simulink model "mpc1_simulation"  (R2022b)
settings: Solver=VariableStepAuto  StartTime=0.0  StopTime=T  RelTol=1e-5
undefined symbols (not defined in the file): Am, Bm, c_1, c_2, C_hilf, Cm, D, dt, F1, H1, PhiU1, PhiZ1, Qy1
settings Model: Creator=benja  LastModifiedBy=benja

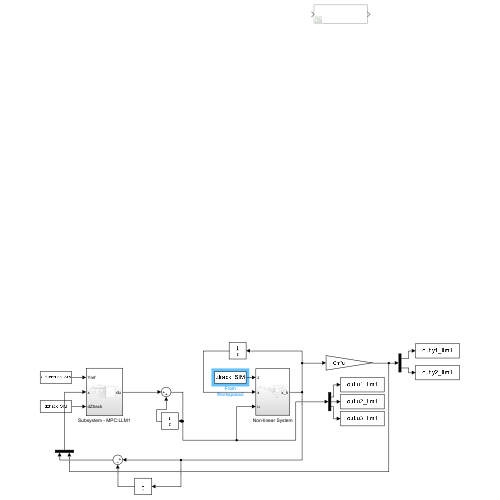
[thumbnail: Simulink's stored preview of the top-level diagram]
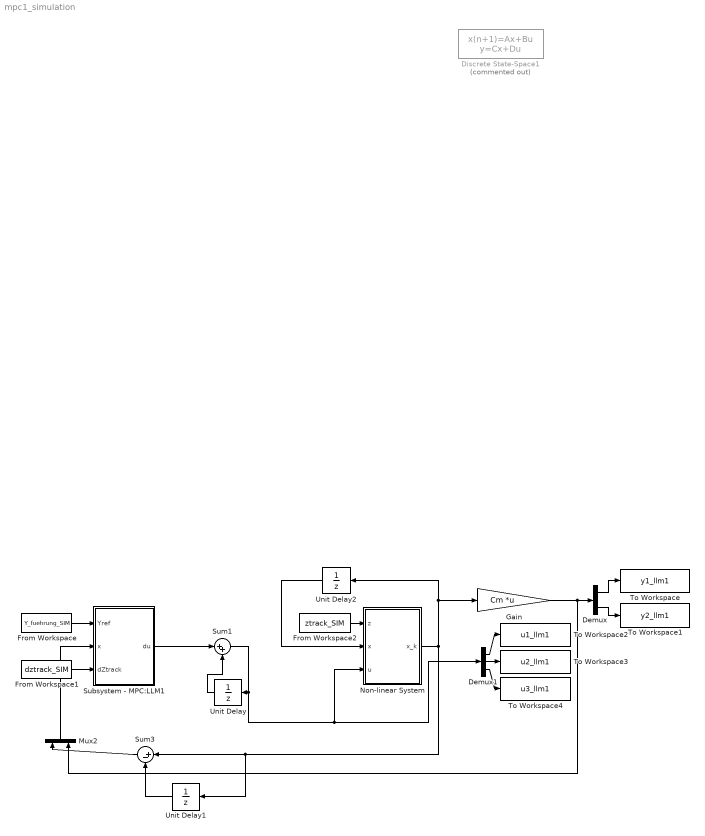
== system mpc1_simulation ==
  Demux : Demux  Outputs=2
  Demux1 : Demux  Outputs=3
  Discrete State-Space1 : DiscreteStateSpace  Commented=on  A=Am  B=Bm  C=C_hilf  D=D  SampleTime=dt
  From Workspace : FromWorkspace  VariableName=Y_fuehrung_SIM  OutDataTypeStr=double  SampleTime=dt
  From Workspace1 : FromWorkspace  VariableName=dztrack_SIM  OutDataTypeStr=double  SampleTime=dt
  From Workspace2 : FromWorkspace  VariableName=ztrack_SIM  OutDataTypeStr=double  SampleTime=dt
  Gain : Gain  Gain=Cm  Multiplication=Matrix(K*u)
  Mux2 : Mux  Inputs=2
  Non-linear System : Subsystem
  Subsystem - MPC:LLM1 : Subsystem
  Sum1 : Sum  Inputs=|++
  Sum3 : Sum  Inputs=|+-
  To Workspace : ToWorkspace  VariableName=y1_llm1  SampleTime=-1
      settings: Save2DSignal=2-D array (concatenate along first dimension)
  To Workspace1 : ToWorkspace  VariableName=y2_llm1  SampleTime=-1
      settings: Save2DSignal=2-D array (concatenate along first dimension)
  To Workspace2 : ToWorkspace  VariableName=u1_llm1  SampleTime=-1
      settings: Save2DSignal=2-D array (concatenate along first dimension)
  To Workspace3 : ToWorkspace  VariableName=u2_llm1  SampleTime=-1
      settings: Save2DSignal=2-D array (concatenate along first dimension)
  To Workspace4 : ToWorkspace  VariableName=u3_llm1  SampleTime=-1
      settings: Save2DSignal=2-D array (concatenate along first dimension)
  Unit Delay : UnitDelay  SampleTime=dt  HasFrameUpgradeWarning=on
  Unit Delay1 : UnitDelay  SampleTime=-1  HasFrameUpgradeWarning=on
  Unit Delay2 : UnitDelay  SampleTime=-1  HasFrameUpgradeWarning=on
  wires:
  Demux/1 -> To Workspace/1
  Demux1/1 -> To Workspace2/1
  Demux1/2 -> To Workspace3/1
  Unit Delay1/1 -> Sum3/2
  Gain/1 -> Demux/1, Mux2/2
  Sum3/1 -> Mux2/1
  Demux1/3 -> To Workspace4/1
  Non-linear System/1(x_k) -> Unit Delay2/1, Gain/1, Unit Delay1/1, Sum3/1
  From Workspace2/1 -> Non-linear System/1(z)
  Unit Delay2/1 -> Non-linear System/2(x)
  Sum1/1 -> Unit Delay/1, Demux1/1, Non-linear System/3(u)
  From Workspace/1 -> Subsystem - MPC:LLM1/1(Yref)
  Mux2/1 -> Subsystem - MPC:LLM1/2(x)
  Demux/2 -> To Workspace1/1
  Unit Delay/1 -> Sum1/2
  From Workspace1/1 -> Subsystem - MPC:LLM1/3(dZtrack)
  Subsystem - MPC:LLM1/1(du) -> Sum1/1

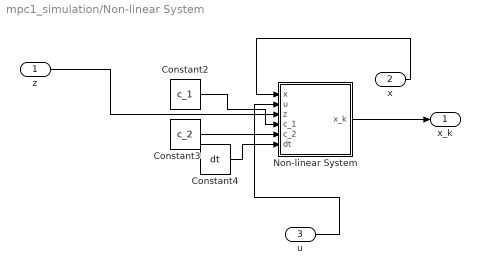
== system mpc1_simulation/Non-linear System ==
  z : Inport
  x : Inport  Port=2
  u : Inport  Port=3
  Constant2 : Constant  Value=c_1
  Constant3 : Constant  Value=c_2
  Constant4 : Constant  Value=dt
  Non-linear System : MATLAB Function  TreatAsAtomicUnit=on
  x_k : Outport
  wires:
  x/1 -> Non-linear System/1(x)
  Constant3/1 -> Non-linear System/5(c_2)
  Constant4/1 -> Non-linear System/6(dt)
  u/1 -> Non-linear System/2(u)
  Constant2/1 -> Non-linear System/4(c_1)
  z/1 -> Non-linear System/3(z)
  Non-linear System/1(x_k) -> x_k/1

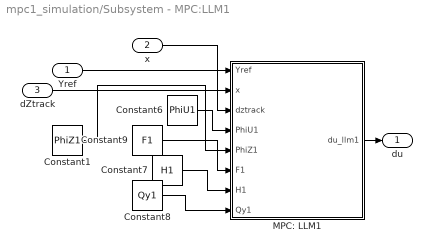
== system mpc1_simulation/Subsystem - MPC:LLM1 ==
  Yref : Inport
  x : Inport  Port=2
  dZtrack : Inport  Port=3
  Constant1 : Constant  Value=PhiZ1  SampleTime=dt
  Constant6 : Constant  Value=PhiU1  SampleTime=dt
  Constant7 : Constant  Value=H1  SampleTime=dt
  Constant8 : Constant  Value=Qy1  SampleTime=dt
  Constant9 : Constant  Value=F1  SampleTime=dt
  MPC: LLM1 : MATLAB Function  TreatAsAtomicUnit=on
  du : Outport
  wires:
  Constant7/1 -> MPC: LLM1/7(H1)
  Constant9/1 -> MPC: LLM1/6(F1)
  x/1 -> MPC: LLM1/2(x)
  Yref/1 -> MPC: LLM1/1(Yref)
  MPC: LLM1/1(du_llm1) -> du/1
  Constant8/1 -> MPC: LLM1/8(Qy1)
  Constant6/1 -> MPC: LLM1/4(PhiU1)
  Constant1/1 -> MPC: LLM1/5(PhiZ1)
  dZtrack/1 -> MPC: LLM1/3(dztrack)

== matlab function mpc1_simulation/Non-linear System/Non-linear System ==
  data: x input size=[4 1]; u input size=[3 1]; z input size=1; x_k output size=[4 1]; c_1 input size=1; c_2 input size=1; dt input size=1
function x_k = fcn(x,u,z,c_1,c_2,dt)
    
    g_RS = 2.6;   
    r_3  = 0.3;   
    r_2 = r_3 / g_RS;    
    r_1 = (r_2 + r_3)/2; 
    r_p = r_3-r_2;
    r_Wheel=0.3;
    g_TT = 66/54*80/23;

    d_s  = 0.096;
    m_p  = 1*4;    
    m_car = 1300;

    J_1  = .1;      
    J_2  = 0.03;     
    J_3  = 0.1;     
    J_p  = 0.01*4;   
    J_4  = m_car*r_Wheel^2 / g_TT^2;  

    M_1 = J_1 + J_2 * 4 * r_1^2/r_2^2 + J_p * r_1^2/r_p^2 + m_p * r_1^2;
    M_2 = J_2 * 2 * r_1 * r_3 / r_2^2 + J_p * r_1 * r_3 / r_p^2;
    M_4 = J_2 * r_3^2 / r_2^2 + J_3 + J_p * r_3^2 / r_p^2;
    M_3 = J_2 * ( (2 * r_1 * r_3 ) / r_2 ^ 2 ) + J_p*((r_1 * r_3) / r_p^2);
    M_5 = M_4 - M_2*M_3/M_1;
    
%     x_k1 = x(3) - x(4);
%     
%     x_k2 = -(M_2/(M_5*M_1)) * ...
%         (c_1*x(4)^2+c_2)*x(1) ... 
%         - (M_2/(M_5*M_1))*d_s*x(3) ...
%         + (M_2/(M_5*M_1))*d_s*x(4) ...
%         + (1+((M_2*M_3)/(M_1*M_5)))/M_1*u(1) ...
%         + ((2*r_1/r_2) + (M_2/M_5)*(2*r_1*M_3/(r_2*M_1) - (r_3/r_2)))/M_1 * u(2) ...
%         + M_2/(M_5*M_1)*u(3);
%     
%     x_k3 = -(1/M_5)*(c_1*x(4)^2+c_2)*x(1)...
%         - (1/M_5)*d_s*x(3) + (1/M_5)*d_s*x(4) + ...
%         M_3/(M_1*M_5)*u(1) + ((2*r_1 * M_3)/(r_2*M_1)-r_3/r_2)/M_5*u(2) + (1/M_5) * u(3); 
%     
%     x_k4 = (1/J_4)*(c_1*x(4)^2+c_2)*x(1) ... 
%         + (1/J_4)*(d_s)*x(3) - (1/J_4)*(d_s) * x(4) - (1/J_4) * z;
% 
%     x_k = x + [x_k1;x_k2;x_k3;x_k4]*dt;
% 


 
    k11 = x(3) - x(4);

    k12 = -(M_2 / (M_5 * M_1)) * (c_1 * x(4)^2 + c_2)*x(1) ...
        - (M_2 / (M_5 * M_1)) * d_s * x(3) ...
        + (M_2 / (M_5 * M_1)) * d_s * x(4) ...
        + (1 + ((M_2 * M_3) / (M_1 * M_5))) * u(1) ...
        + ((2 * r_1 / r_2) + (M_2 / M_5) * (2 *r_1 * M_3 / (r_2 * M_1) - (r_3 / r_2))) / M_1 * u(2) ...
        + M_2 / (M_5 * M_1) * u(3);
    
    k13 = -(1 / M_5) * (c_1 * x(4)^2 + c_2) * x(1) - (1 / M_5) * d_s * x(3) + (1 / M_5) * d_s * x(4) + ...
        M_3 / (M_1 * M_5) * u(1) + ((2 * r_1 * M_3) / (r_2 * M_1) - r_3 / r_2) / M_5 * u(2) + (1 / M_5) * u(3);

    k14 = (1 / J_4) * (c_1 * x(4)^2 + c_2) * x(1) + (1 / J_4)*(d_s) * x(3) - ( 1 / J_4) * (d_s) * x(4) - (1 / J_4) * z;
 

    k21 = (x(3) + k13 * dt / 2) - (x(4) + k14 * dt / 2);

    k22 = -(M_2 / (M_5 * M_1)) * (c_1 * (x(4) + k14 * dt / 2)^2 + c_2) * (x(1) + k11 * dt / 2) ...
        - (M_2 / (M_5 * M_1)) * d_s * (x(3) + k13 * dt / 2) ...
        + (M_2 / (M_5 * M_1)) * d_s * (x(4) + k14 * dt / 2) ...
        + (1+ ((M_2 * M_3) / (M_1 * M_5))) * u(1) ...
        + ((2 * r_1 / r_2) + (M_2 / M_5) * ( 2 * r_1 * M_3 / (r_2 * M_1) - (r_3 / r_2))) / M_1 * u(2) ...
        + M_2 / (M_5 * M_1) * u(3);
        
    k23 = -(1 / M_5) * (c_1 * (x(4) + k14 * dt / 2)^2+c_2)*(x(1) + k11 * dt / 2) ...
        - (1 / M_5) * d_s * (x(3) + k13 * dt / 2) ...
        + (1 / M_5) * d_s * ( x(4) + k14 * dt / 2) ...
        + M_3 / (M_1 * M_5) * u(1) ...
        + ((2 * r_1 * M_3) / (r_2 * M_1) - r_3 / r_2) / M_5 * u(2) ...
        + (1 / M_5) * u(3);
    
    k24 = (1 / J_4) * (c_1 * (x(4) + k14 * dt / 2)^2 + c_2)*(x(1) + k11 * dt / 2) ...
        + (1 / J_4) * (d_s) * (x(3) + k13 * dt / 2) ...
        - (1 / J_4) * (d_s) * (x(4) + k14 * dt / 2) ...
        - (1 / J_4) * z;
   

    k31 = (x(3) + k23 * dt / 2) - (x(4) + k24 * dt / 2);

    k32 = -(M_2 / (M_5 * M_1)) * (c_1 * (x(4) + k24 * dt / 2)^2 + c_2) * (x(1) + k21 * dt / 2) ...
        - (M_2 / (M_5 * M_1)) * d_s * (x(3) + k23 * dt / 2) ...
        + (M_2 / (M_5 * M_1)) * d_s * (x(4) + k24 * dt / 2) ...
        + (1 + ((M_2 * M_3) / (M_1 * M_5))) * u(1) ...
        + ((2 * r_1 / r_2) + (M_2 / M_5) * (2 * r_1 * M_3 / (r_2 * M_1) - (r_3 / r_2))) / M_1 * u(2) ...
        + M_2 / (M_5 * M_1) * u(3);
    
    k33 = -(1 / M_5)*(c_1 * (x(4) + k24 * dt / 2)^2 + c_2) * (x(1) + k21 * dt / 2) ...
        - (1 / M_5) * d_s * (x(3) + k23 * dt / 2) ...
        + (1 / M_5) * d_s * (x(4) + k24 * dt / 2) ...
        + M_3 / (M_1 * M_5) * u(1) ...
        + ((2 * r_1 * M_3) / (r_2 * M_1) - r_3 / r_2) / M_5 * u(2) ...
        + (1 / M_5) * u(3);
    
    k34 = (1 / J_4) * (c_1 * (x(4) + k24 * dt / 2)^2 + c_2) * (x(1) + k21 * dt / 2) ...
        + (1 / J_4) * (d_s) * (x(3) + k23 * dt /2) ...
        - (1 / J_4) * (d_s) * (x(4) + k24 * dt / 2) ...
        - (1 / J_4) * z;
    

    k41 = (x(3) + k33 * dt) - (x(4) + k34 * dt);

    k42 = -(M_2 / (M_5 * M_1)) * (c_1 * (x(4) + k34 * dt)^2 + c_2) * (x(1) + k31 * dt) ...
        - (M_2 / (M_5 * M_1)) * d_s * (x(3) + k33 * dt ) ...
        + (M_2 / (M_5 * M_1)) * d_s * (x(4) + k34 * dt ) ...
        + (1 + ((M_2 * M_3) / (M_1 * M_5))) * u(1) ...
        + ((2 * r_1 / r_2) + (M_2 / M_5) * (2 * r_1 * M_3 / (r_2 * M_1) - (r_3 / r_2))) / M_1 * u(2) ...
        + M_2 / (M_5 * M_1) * u(3);
    
    k43 = -(1 / M_5) * (c_1 * (x(4) + k34 * dt)^2 + c_2) * (x(1) + k31 * dt ) ...
        - (1 / M_5) * d_s * (x(3) + k33 * dt ) ...
        + (1 / M_5) * d_s * (x(4) + k34 * dt ) ...
        + M_3 / (M_1 * M_5) * u(1) ...
        + ((2 * r_1 * M_3)/(r_2 * M_1) - r_3 / r_2) / M_5 * u(2) ...
        + (1 / M_5) * u(3);
    
    k44 = (1 / J_4) * (c_1 * (x(4) + k34 * dt )^2 + c_2) * (x(1) + k31 * dt ) ...
        + (1 / J_4) * (d_s) * (x(3) + k33 * dt ) ...
        - (1 / J_4) * (d_s) * (x(4) + k34 * dt ) ...
        - (1 / J_4) * z;

    x_k = x + dt * ([k11;k12;k13;k14] + 2 * [k21;k22;k23;k24] + 2 * [k31;k32;k33;k34] + [k41;k42;k43;k44]) / 6;

== matlab function mpc1_simulation/Subsystem - MPC:LLM1/MPC: LLM1 ==
  data: Yref input size=[100 1]; du_llm1 output size=[3 1]; x input size=[6 1]; dztrack input size=[50 1]; PhiU1 input size=[100 45]; PhiZ1 input size=[100 50]; F1 input size=[100 6]; H1 input size=[45 45]; Qy1 input size=[100 100]
function du_llm1 = fcn(Yref,x,dztrack,PhiU1,PhiZ1,F1,H1,Qy1)
    nu = 3;
    f = -PhiU1' * Qy1 * ( Yref - F1*x - PhiZ1*dztrack);
    dU = -H1\f; % -inv(H)*f
    du_llm1 = dU(1:nu,1);
    
end
